simulink model "mconversion13"  (Simulink 6.0)
settings: Solver=FixedStepDiscrete  StartTime=0.0  StopTime=10.0  RelTol=1e-3
settings Model: Creator=myunt  LastModifiedBy=myunt  ExtModeAutoUpdateStatusClock=off
settings DebuggingCC: CheckExecutionContextPreStartOutputMsg=on  CheckExecutionContextRuntimeOutputMsg=on

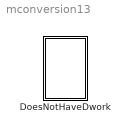
== system mconversion13 ==
  DoesNotHaveDwork : Subsystem  TreatAsAtomicUnit=on  PropExecContextAcrossSSBoundary=on

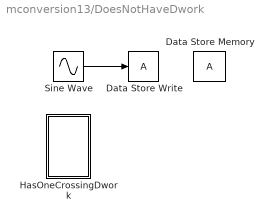
== system mconversion13/DoesNotHaveDwork ==
  Data Store Memory : DataStoreMemory  DialogController=Simulink.DDGSource  DataStoreName=A  InitialValue=0
  Data Store Write : DataStoreWrite  DialogController=Simulink.DDGSource  DataStoreName=A  SampleTime=-1
  HasOneCrossingDwork : Subsystem  TreatAsAtomicUnit=on  PropExecContextAcrossSSBoundary=on
      settings: RTWSystemCode=Function
  Sine Wave : Sin  SampleTime=0
  wires:
  Sine Wave/1 -> Data Store Write/1

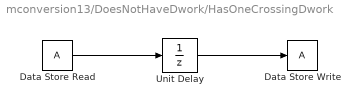
== system mconversion13/DoesNotHaveDwork/HasOneCrossingDwork ==
  Data Store Read : DataStoreRead  DialogController=Simulink.DDGSource  DataStoreName=A  SampleTime=0
  Data Store Write : DataStoreWrite  DialogController=Simulink.DDGSource  DataStoreName=A  SampleTime=-1
  Unit Delay : UnitDelay
  wires:
  Data Store Read/1 -> Unit Delay/1
  Unit Delay/1 -> Data Store Write/1
